simulink model "Inicializar2"  (R2023b)
settings: Solver=VariableStepAuto  StartTime=0.0  StopTime=20  RelTol=1e-3
settings Model: Creator=LENOVO  LastModifiedBy=LENOVO

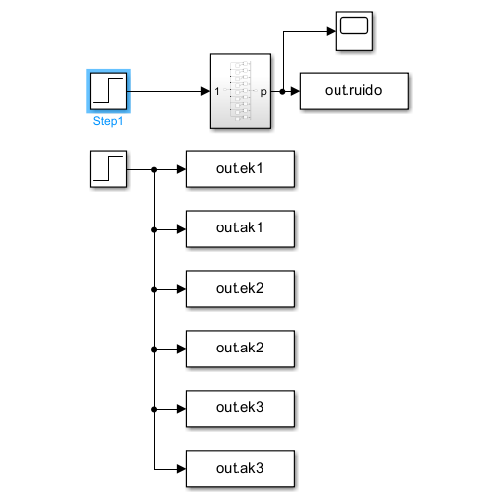
[thumbnail: Simulink's stored preview of the top-level diagram]
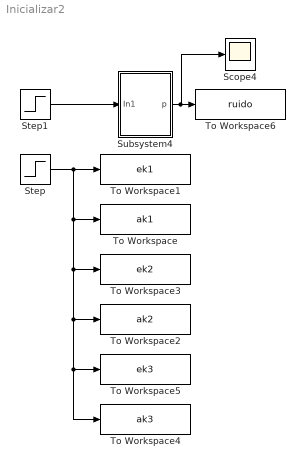
== system Inicializar2 ==
  Scope4 : Scope
  Step : Step  After=0  SampleTime=0
  Step1 : Step  Time=0  After=0.8  SampleTime=0
  Subsystem4 : Subsystem
  To Workspace : ToWorkspace  VariableName=ak1  SampleTime=-1
  To Workspace1 : ToWorkspace  VariableName=ek1  SampleTime=-1
  To Workspace2 : ToWorkspace  VariableName=ak2  SampleTime=-1
  To Workspace3 : ToWorkspace  VariableName=ek2  SampleTime=-1
  To Workspace4 : ToWorkspace  VariableName=ak3  SampleTime=-1
  To Workspace5 : ToWorkspace  VariableName=ek3  SampleTime=-1
  To Workspace6 : ToWorkspace  VariableName=ruido  SampleTime=-1
  wires:
  Step1/1 -> Subsystem4/1(In1)
  Subsystem4/1(p) -> Scope4/1, To Workspace6/1
  Step/1 -> To Workspace5/1, To Workspace4/1, To Workspace2/1, To Workspace3/1, To Workspace/1, To Workspace1/1

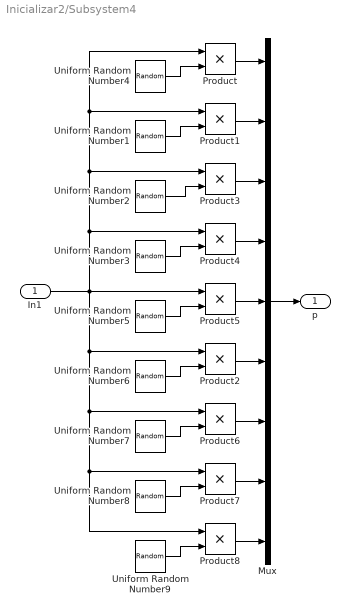
== system Inicializar2/Subsystem4 ==
  In1 : Inport
  Mux : Mux  Inputs=9
  Product{,1..8} (9 alike) : Product
  Uniform Random Number1 : UniformRandomNumber  Minimum=-0.002  Maximum=0.002  Seed=2  SampleTime=0.1
  Uniform Random Number2 : UniformRandomNumber  Minimum=-0.002  Maximum=0.002  Seed=1  SampleTime=0.1
  Uniform Random Number3 : UniformRandomNumber  Minimum=-0.002  Maximum=0.002  Seed=3  SampleTime=0.1
  Uniform Random Number4 : UniformRandomNumber  Minimum=-0.002  Maximum=0.002  SampleTime=0.1
  Uniform Random Number5 : UniformRandomNumber  Minimum=-0.002  Maximum=0.002  Seed=1.5  SampleTime=0.1
  Uniform Random Number6 : UniformRandomNumber  Minimum=-0.002  Maximum=0.002  Seed=3  SampleTime=0.1
  Uniform Random Number7 : UniformRandomNumber  Minimum=-0.002  Maximum=0.002  Seed=1.5  SampleTime=0.1
  Uniform Random Number8 : UniformRandomNumber  Minimum=-0.002  Maximum=0.002  Seed=3  SampleTime=0.1
  Uniform Random Number9 : UniformRandomNumber  Minimum=-0.002  Maximum=0.002  Seed=1.5  SampleTime=0.1
  p : Outport
  wires:
  Product/1 -> Mux/1
  Uniform Random Number5/1 -> Product5/2
  Uniform Random Number1/1 -> Product1/2
  Uniform Random Number2/1 -> Product3/2
  Product4/1 -> Mux/4
  Product1/1 -> Mux/2
  Uniform Random Number3/1 -> Product4/2
  Uniform Random Number4/1 -> Product/2
  Product3/1 -> Mux/3
  Product5/1 -> Mux/5
  Mux/1 -> p/1
  Uniform Random Number7/1 -> Product6/2
  Uniform Random Number6/1 -> Product2/2
  Uniform Random Number8/1 -> Product7/2
  In1/1 -> Product3/1, Product/1, Product1/1, Product4/1, Product2/1, Product7/1, Product8/1, Product6/1, Product5/1
  Uniform Random Number9/1 -> Product8/2
  Product8/1 -> Mux/9
  Product2/1 -> Mux/6
  Product6/1 -> Mux/7
  Product7/1 -> Mux/8
